simulink model "sin_wave"  (R2023b)
settings: Solver=VariableStepAuto  StartTime=0.0  StopTime=10.0  MaxStep=0.01  RelTol=1e-3

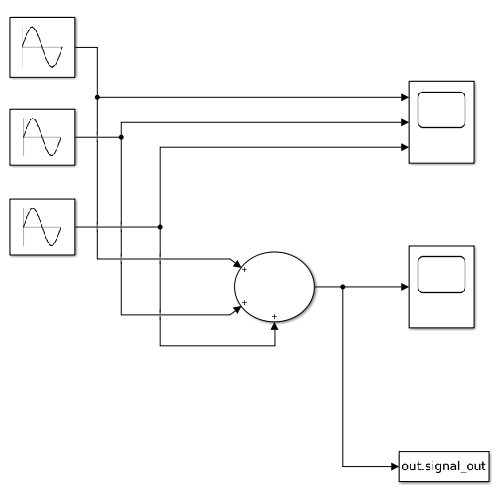
[thumbnail: Simulink's stored preview of the top-level diagram]
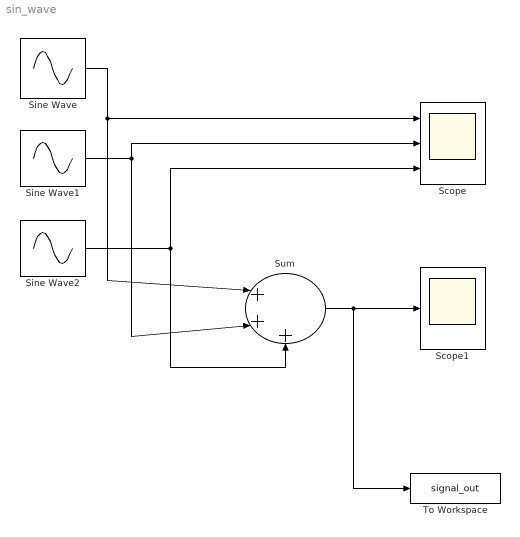
== system sin_wave ==
  Scope : Scope  NumInputPorts=3
  Scope1 : Scope
  Sine Wave : Sin  Amplitude=3  SampleTime=0
  Sine Wave1 : Sin  Amplitude=5  Frequency=5  SampleTime=0
  Sine Wave2 : Sin  Amplitude=10  Frequency=10  SampleTime=0
  Sum : Sum  Inputs=|+++
  To Workspace : ToWorkspace  VariableName=signal_out  SaveFormat=Timeseries  SampleTime=-1
  wires:
  Sine Wave/1 -> Scope/1, Sum/1
  Sine Wave1/1 -> Scope/2, Sum/2
  Sine Wave2/1 -> Scope/3, Sum/3
  Sum/1 -> To Workspace/1, Scope1/1
